simulink model "tested"  (R2014a)
settings: Solver=ode45  StartTime=0.0  StopTime=100.0  RelTol=1e-3
settings Model: Creator=eliasseb  LastModifiedBy=eliasseb

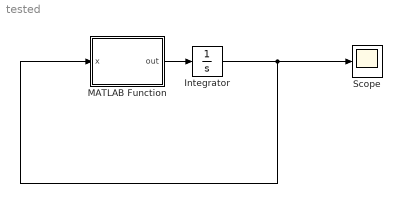
== system tested ==
  Integrator : Integrator
  MATLAB Function : MATLAB Function  TreatAsAtomicUnit=on
  Scope : Scope
  wires:
  MATLAB Function/1(out) -> Integrator/1
  Integrator/1 -> MATLAB Function/1(x), Scope/1

== matlab function tested/MATLAB Function ==
  data: x input; out output
function out   = tester( x )
%UNTITLED Summary of this function goes here
%   Detailed explanation goes here
%#codegen
ref=1;
 h=0.1;

out=-(x-ref)*h;

end
